simulink model "wheels2fin"  (R2014a)
settings: Solver=ode15s  StartTime=0.0  StopTime=20  MaxStep=.01  RelTol=1e-3  AbsTol=1e-6  EnableMultiTasking=on
PreLoadFcn:
  | % Load initialization data
  | 
  | sldemo_absdata;
StopFcn:
  | if exist ('wheels2_output')
  |   wheels2plots;
  | end
undefined symbols (not defined in the file): ctrl, mu, slip
libraries: fl_lib x5, sh_lib x3, nesl_utility x3, aerospace x1, powerlib_meascontrol x1, simulink x1
CloseFcn:
  | % Close the plots that are still open
  | h = findobj(0, 'Name', 'ABS Speeds');
  | if ~isempty(h),
  |   close(h);
  | end;
  | 
  | h = findobj(0, 'Name', 'ABS Slip');
  | if ~isempty(h),
  |   close(h);
  | end;
  | 
  | % Clear initial conditions data to avoid cluttering the workspace
  | 
  | clear g v0 Rr Kf m PBmax TB I slip mu ctrl h;
Description:
  | Modeling an Anti-Lock Braking System (ABS)
  | 
  | *Summary*
  | 
  | This example describes a simple model for an Anti-Lock Braking System
  | (ABS). The model simulates the dynamic behavior of a vehicle
  | under hard braking conditions. The model represents a single wheel, which
  | may be replicated a number of times to create a model for a multi-wheel
  | vehicle.
  | 
  | This model uses the signal logging feature in Simulink(R). You log signals to the
  | MATLAB(R) workspace where you can analyze and view them. You can view
  | the code in sldemo_absbrakeplots.m to see how this is done.
  | 
  | In this model, the wheel speed is calculated in a separate component
  | named sldemo_wheelspeed_absbrake.
  | This component is then referenced using a Model block.  Note that both the
  | top model and the referenced model use a variable step solver, so Simulink
  | will track zero-crossings in the referenced model.
settings Model: FPTRunName=Active  ExtModeTrigMode=oneshot  ExtModeTrigDuration=8  ExtModeArmWhenConnect=off  ExtModeAutoUpdateStatusClock=off  Creator=The MathWorks, Inc.  LastModifiedBy=Abi
settings SolverCC: AutoScaleAbsTol=off
settings DataIOCC: LimitDataPoints=off  SaveOutput=off  SaveTime=off  TimeSaveName=time  SignalLoggingName=sldemo_absbrake_output
settings OptimizationCC: DefaultUnderspecifiedDataType=single  EnhancedBackFolding=on  PassReuseOutputArgsAs=Individual arguments  ExpressionDepthLimit=2147483647  InitFltsAndDblsToZero=on  LifeSpan=auto  MaxStackSize=512  BufferReusableBoundary=off  SimCompilerOptimization=off  OptimizeBlockOrder=speed  DifferentSizesBufferReuse=on  OptimizationCustomize=off
settings DebuggingCC: SaveWithParameterizedLinksMsg=none  MergeDetectMultiDrivingBlocksExec=error  SolverPrmCheckMsg=none  MultiTaskDSMMsg=warning  SigSpecEnsureSampleTimeMsg=none  IntegerOverflowMsg=none  ParameterTunabilityLossMsg=error  FcnCallInpInsideContextMsg=warning  FrameProcessingCompatibilityMsg=error  BusObjectLabelMismatch=none  AllowSymbolicDim=off  StateNameClashWarn=warning  SFExecutionAtInitializationDiag=none  IntegerSaturationMsg=none  ArithmeticOperatorsInVariantConditions=warning
settings HardwareCC: ProdBitPerChar=16  ProdBitPerInt=16  ProdBitPerSizeT=32  ProdBitPerPtrDiffT=32  ProdLargestAtomicInteger=Integer  ProdIntDivRoundTo=Zero  ProdEndianess=LittleEndian  ProdWordSize=16  ProdLongLongMode=on  ProdHWDeviceType=Texas Instruments->C2000  TargetBitPerPointer=64  TargetBitPerSizeT=64  TargetBitPerPtrDiffT=64  TargetLongLongMode=on  TargetIntDivRoundTo=Zero  TargetEndianess=LittleEndian  TargetWordSize=64  TargetHWDeviceType=MATLAB Host
settings ModelReferenceCC: UpdateModelReferenceTargets=IfOutOfDate
settings SFSimCC: MATLABDynamicMemAlloc=off
settings RTWCC: SystemTargetFile=ert.tlc  HardwareBoard=TI Piccolo F28069M LaunchPad  TLCOptions=-aInlineSetEventsForThisBaseRateFcn=TLC_FALSE -aSuppressMultiTaskScheduler=TLC_FALSE -aRateBasedStepFcn=1  TemplateMakefile=ert_default_tmf  Description=Embedded Coder  GenerateReport=on  Toolchain=Texas Instruments Code Composer Studio (C2000)  IncludeHyperlinkInReport=on  LaunchReport=on  GenerateTraceInfo=on  GenerateTraceReport=on  GenerateTraceReportSl=on  GenerateTraceReportSf=on  GenerateTraceReportEml=on  RTWCompilerOptimization=off
settings CodeAppCC: ForceParamTrailComments=on  IgnoreCustomStorageClasses=off  OperatorAnnotations=on  SimulinkDataObjDesc=on  SFDataObjDesc=on  InsertBlockDesc=on
settings ERTTargetCC: CodeReplacementLibrary=TI C28x  MultiwordLength=256  GenerateSampleERTMain=off  ParMdlRefBuildCompliant=on  CompOptLevelCompliant=on  ConcurrentExecutionCompliant=on  ModelStepFunctionPrototypeControlCompliant=on  CPPClassGenCompliant=on  InlinedParameterPlacement=Hierarchical  ConvertIfToSwitch=on  SuppressUnreachableDefaultCases=on
settings ConfigComp: CovMetricSettings=dw  CovHtmlReporting=on  CovSaveCumulativeToWorkspaceVar=on  CovSaveSingleToWorkspaceVar=on  CovExternalEMLEnable=off  CovSFcnEnable=off

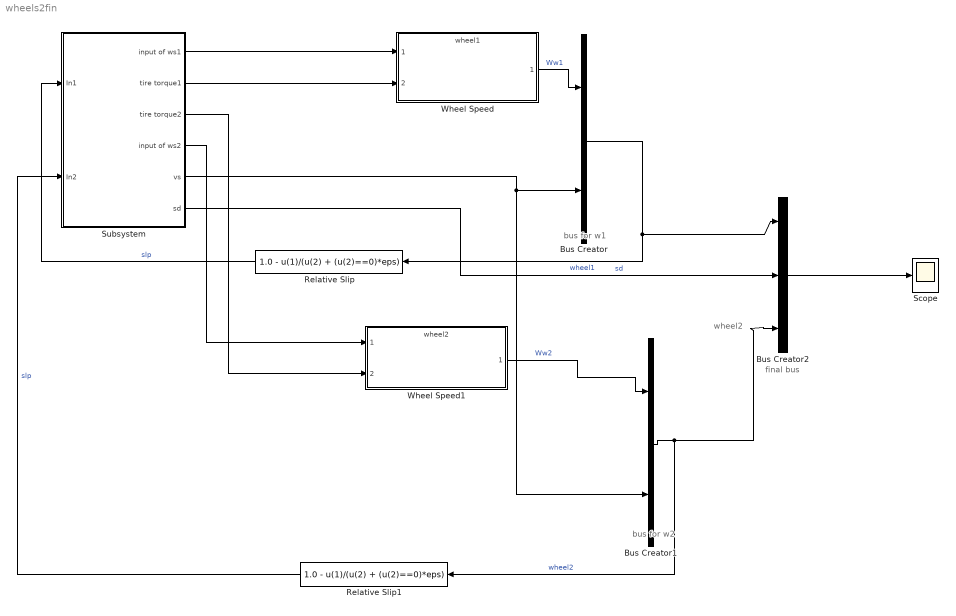
== system wheels2fin ==
  note: bus for w2
  note: bus for w1
  note: final bus
  note: wheel2
  Bus Creator2 : BusCreator  Inputs=3
  Bus Creator : BusCreator  Inputs=2
  Bus Creator1 : BusCreator  Inputs=2
  Relative Slip : Fcn  Expr=1.0 - u(1)/(u(2) + (u(2)==0)*eps)
  Relative Slip1 : Fcn  Expr=1.0 - u(1)/(u(2) + (u(2)==0)*eps)
  Scope : Scope
  Subsystem : Subsystem
  Wheel Speed : ModelReference  ModelNameDialog=wheel1.slx  SimulationMode=Normal  ModelReferenceVersion=1.65  CopyOfModelName=wheel1.slx  DefaultDataLogging=on
  Wheel Speed1 : ModelReference  ModelNameDialog=wheel2.slx  SimulationMode=Normal  ModelReferenceVersion=1.65  CopyOfModelName=wheel2.slx  DefaultDataLogging=on
  wires:
  Wheel Speed/1 -> Bus Creator/1  "Ww1"
  Relative Slip/1 -> Subsystem/1(In1)  "slp"
  Bus Creator/1 -> Relative Slip/1, Bus Creator2/1  "wheel1"
  Wheel Speed1/1 -> Bus Creator1/1  "Ww2"
  Bus Creator1/1 -> Bus Creator2/3, Relative Slip1/1  "wheel2"
  Relative Slip1/1 -> Subsystem/2(In2)  "slp"
  Subsystem/1(input of ws1) -> Wheel Speed/1
  Subsystem/2("tire torque1 ") -> Wheel Speed/2
  Subsystem/3(tire torque2) -> Wheel Speed1/2
  Subsystem/5(vs) -> Bus Creator1/2, Bus Creator/2
  Subsystem/4(input of ws2) -> Wheel Speed1/1
  Bus Creator2/1 -> Scope/1
  Subsystem/6("sd ") -> Bus Creator2/2  "sd"

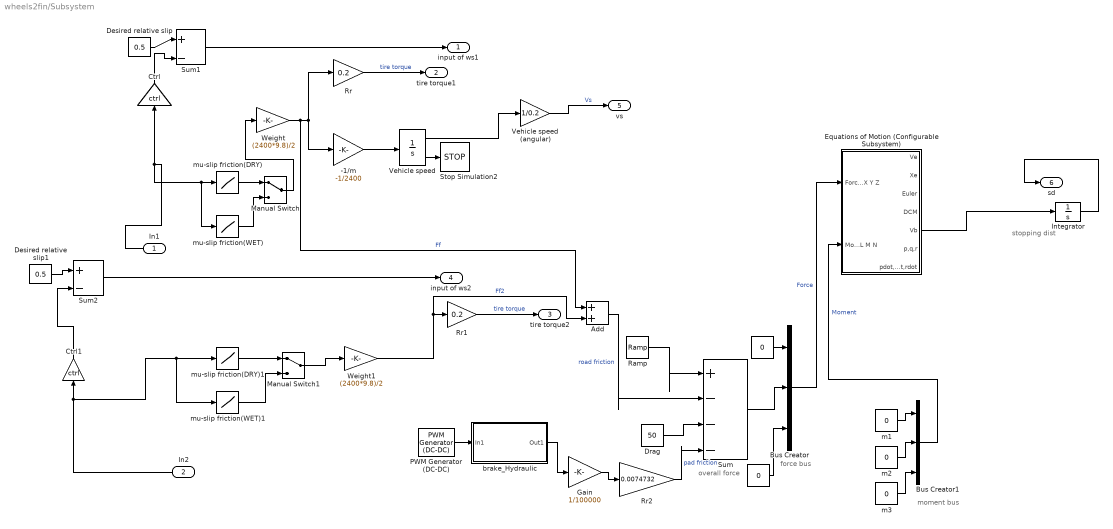
== system wheels2fin/Subsystem ==
  note: moment bus
  note: force bus
  note: stopping dist
  note: overall force
  In1 : Inport
  In2 : Inport  Port=2
  " " : Constant  Value=0
  " " : Constant  Value=0
  -1/m : Gain  Gain=-1/2400  SaturateOnIntegerOverflow=on  OutDataTypeStr=Inherit: Same as input  ParamDataTypeStr=Inherit: Same as input
  Add : Sum
  Bus Creator : BusCreator  Inputs=3
  Bus Creator1 : BusCreator  Inputs=3
  Ctrl : Gain  Gain=ctrl  SaturateOnIntegerOverflow=on  OutDataTypeStr=Inherit: Same as input  ParamDataTypeStr=Inherit: Same as input
  Ctrl1 : Gain  Gain=ctrl  SaturateOnIntegerOverflow=on  OutDataTypeStr=Inherit: Same as input  ParamDataTypeStr=Inherit: Same as input
  Desired relative slip : Constant  Value=0.5
  Desired relative slip1 : Constant  Value=0.5
  Drag : Constant  Value=50
  Equations of Motion (Configurable Subsystem) : Subsystem  BlockChoice=Euler Angles
      link override Euler Angles: Mass=2400
      settings: AttributesFormatString=%<BlockChoice>  MemberBlocks=Euler Angles,Quaternions
      settings: TemplateBlock=|
      | aerospace/6DoF/Equations of Motion
      | (Configurable Subsystem)
  Gain : Gain  Gain=1/100000
  Integrator : Integrator
  Manual Switch : ManualSwitch
  Manual Switch1 : ManualSwitch
  PWM Generator (DC-DC) : powerlib_meascontrol/Pulse & Signal Generators/PWM Generator (DC-DC)  Fsw=5000  Ts=0
  Ramp : simulink/Sources/Ramp  slope=1  start=0  X0=0
  Rr : Gain  Gain=0.2  SaturateOnIntegerOverflow=on  OutDataTypeStr=Inherit: Same as input  ParamDataTypeStr=Inherit: Same as input
  Rr1 : Gain  Gain=0.2  SaturateOnIntegerOverflow=on  OutDataTypeStr=Inherit: Same as input  ParamDataTypeStr=Inherit: Same as input
  Rr2 : Gain  Gain=0.0074732  SaturateOnIntegerOverflow=on  OutDataTypeStr=Inherit: Same as input  ParamDataTypeStr=Inherit: Same as input
  Stop Simulation2 : Stop
  Sum : Sum  Inputs=|+---
  Sum1 : Sum  Inputs=|+-  SaturateOnIntegerOverflow=on  InputSameDT=on  OutDataTypeStr=Inherit: Same as first input
  Sum2 : Sum  Inputs=|+-  SaturateOnIntegerOverflow=on  InputSameDT=on  OutDataTypeStr=Inherit: Same as first input
  Vehicle speed : Integrator  UpperSaturationLimit=1000  LowerSaturationLimit=0  ShowSaturationPort=on
  Vehicle speed (angular) : Gain  Gain=1/0.2  SaturateOnIntegerOverflow=on  OutDataTypeStr=Inherit: Same as input  ParamDataTypeStr=Inherit: Same as input
  Weight : Gain  Gain=(2400*9.8)/2  SaturateOnIntegerOverflow=on  OutDataTypeStr=Inherit: Same as input  ParamDataTypeStr=Inherit: Same as input
  Weight1 : Gain  Gain=(2400*9.8)/2  SaturateOnIntegerOverflow=on  OutDataTypeStr=Inherit: Same as input  ParamDataTypeStr=Inherit: Same as input
  "brake_Hydraulic " : Subsystem
  m1 : Constant  Value=0
  "m2 " : Constant  Value=0
  m3 : Constant  Value=0
  mu-slip friction(DRY) : Lookup_n-D  NumberOfTableDimensions=1  BreakpointsForDimension1=slip  Table=mu  SaturateOnIntegerOverflow=on  InputSameDT=on
  mu-slip friction(DRY)1 : Lookup_n-D  NumberOfTableDimensions=1  BreakpointsForDimension1=slip  Table=mu  SaturateOnIntegerOverflow=on  InputSameDT=on
  mu-slip friction(WET) : Lookup_n-D  NumberOfTableDimensions=1  BreakpointsForDimension1=slip  Table=mu  SaturateOnIntegerOverflow=on  InputSameDT=on
  mu-slip friction(WET)1 : Lookup_n-D  NumberOfTableDimensions=1  BreakpointsForDimension1=slip  Table=mu  SaturateOnIntegerOverflow=on  InputSameDT=on
  input of ws1 : Outport
  "tire torque1 " : Outport  Port=2
  tire torque2 : Outport  Port=3
  input of ws2 : Outport  Port=4
  vs : Outport  Port=5
  "sd " : Outport  Port=6
  wires:
  Weight/1 -> Add/1, -1/m/1, Rr/1  "Ff"
  Rr/1 -> "tire torque1 "/1  "tire torque"
  Sum1/1 -> input of ws1/1
  -1/m/1 -> Vehicle speed/1
  Desired relative slip/1 -> Sum1/1
  Ctrl/1 -> Sum1/2
  Vehicle speed/2 -> Stop Simulation2/1
  Vehicle speed/1 -> Vehicle speed (angular)/1
  Vehicle speed (angular)/1 -> vs/1  "Vs"
  Desired relative slip1/1 -> Sum2/1
  Sum2/1 -> input of ws2/1
  Ctrl1/1 -> Sum2/2
  Rr1/1 -> tire torque2/1  "tire torque"
  Weight1/1 -> Add/2, Rr1/1  "Ff2"
  "brake_Hydraulic "/1(Out1) -> Gain/1
  Ramp/1 -> Sum/1
  Add/1 -> Sum/2  "road friction"
  Drag/1 -> Sum/3
  " "/1 -> Bus Creator/3
  m3/1 -> Bus Creator1/3
  "m2 "/1 -> Bus Creator1/2
  m1/1 -> Bus Creator1/1
  Bus Creator1/1 -> Equations of Motion (Configurable Subsystem)/2(Moments L M N)  "Moment"
  Integrator/1 -> "sd "/1
  Bus Creator/1 -> Equations of Motion (Configurable Subsystem)/1(Forces X Y Z)  "Force"
  Equations of Motion (Configurable Subsystem)/5(Vb) -> Integrator/1
  " "/1 -> Bus Creator/1
  Sum/1 -> Bus Creator/2
  Gain/1 -> Rr2/1
  Rr2/1 -> Sum/4  "pad friction"
  In2/1 -> mu-slip friction(WET)1/1, mu-slip friction(DRY)1/1, Ctrl1/1
  In1/1 -> Ctrl/1, mu-slip friction(WET)/1, mu-slip friction(DRY)/1
  mu-slip friction(DRY)/1 -> Manual Switch/1
  mu-slip friction(WET)/1 -> Manual Switch/2
  Manual Switch/1 -> Weight/1
  mu-slip friction(DRY)1/1 -> Manual Switch1/1
  mu-slip friction(WET)1/1 -> Manual Switch1/2
  Manual Switch1/1 -> Weight1/1
  PWM Generator (DC-DC)/1 -> "brake_Hydraulic "/1(In1)

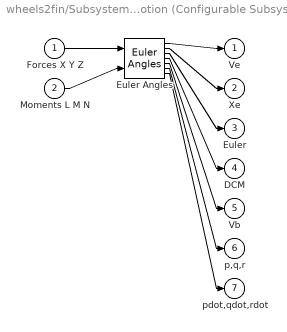
== system wheels2fin/Subsystem/Equations of Motion (Configurable Subsystem) ==
  Forces X Y Z : Inport
  Moments L M N : Inport  Port=2
  Euler Angles : aerospace/6DoF/Euler Angles  xme_0=[0 0 0]  Vm_0=[0 0 0]  eul_0=[0 0 0]  pm_0=[0 0 0]  Mass=2400  Inertia=eye(3)
  Ve : Outport
  Xe : Outport  Port=2
  Euler : Outport  Port=3
  DCM : Outport  Port=4
  Vb : Outport  Port=5
  p,q,r : Outport  Port=6
  pdot,qdot,rdot : Outport  Port=7
  wires:
  Forces X Y Z/1 -> Euler Angles/1
  Moments L M N/1 -> Euler Angles/2
  Euler Angles/1 -> Ve/1
  Euler Angles/2 -> Xe/1
  Euler Angles/3 -> Euler/1
  Euler Angles/4 -> DCM/1
  Euler Angles/5 -> Vb/1
  Euler Angles/6 -> p,q,r/1
  Euler Angles/7 -> pdot,qdot,rdot/1

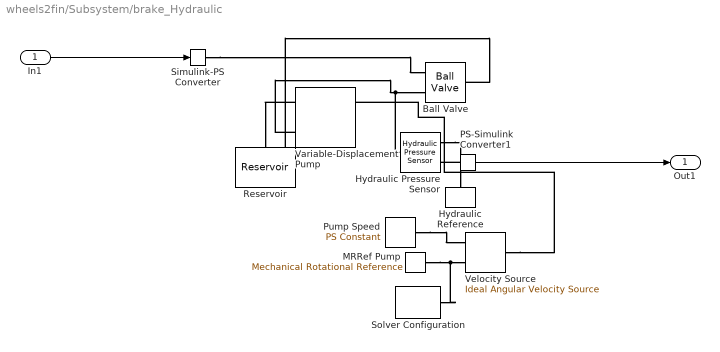
== system wheels2fin/Subsystem/brake_Hydraulic  ==
  In1 : Inport
  Ball Valve : sh_lib/Valves/Flow Control Valves/Ball Valve  d_ball=0.01 m  d_orif=0.005 m  x_0=0 m  C_d=0.65  Re_cr=10  A_leak=1e-12 m^2
  Hydraulic Pressure Sensor : fl_lib/Hydraulic/Hydraulic Sensors/Hydraulic Pressure Sensor
  Hydraulic Reference : fl_lib/Hydraulic/Hydraulic Elements/Hydraulic Reference
  MRRef Pump : fl_lib/Mechanical/Rotational Elements/Mechanical Rotational Reference  Tag=Factory Generic
  PS-Simulink Converter1 : nesl_utility/PS-Simulink Converter  PhysicalDomain=network_engine_domain  SubClassName=ps_output  LeftPortType=input  RightPortType=output  PseudoPeriodic=off  Frequencies=[]  Unit=1  AffineConversion=off
  Pump Speed : fl_lib/Physical Signals/Sources/PS Constant  constant=1
  Reservoir : sh_lib/Hydraulic Utilities/Reservoir  press=0 Pa  init_volume=0.02 m^3  ret_diam=0.02 m  loss_coeff=1  Re_lam=15  area=1e-4 m^2  p_cr=1e-5 Pa
  Simulink-PS Converter : nesl_utility/Simulink-PS Converter  PhysicalDomain=network_engine_domain  SubClassName=ps_input  LeftPortType=input  RightPortType=output  PseudoPeriodic=off  Frequencies=[]  NoiseDistribution=none  NoiseParameters=[]  Unit=1  AffineConversion=off  InputFiltering=off  SimscapeFilterOrder=1  InputFilterTimeConstant=0.001  UdotUserProvided=1
  Solver Configuration : nesl_utility/Solver Configuration  PhysicalDomain=network_engine_domain  SubClassName=solver  LeftPortType=input  RightPortType=generic  Accelerate=off  Tones=[]  Harmonics=[]  SimulateNoise=off  Profile=off  UseLocalSampling=off  EnableSwitchedLinearOptims=on  FrequencyDomain=off  UseCCode=off  RelTol=0.001  AbsTol=1e-06  MinStep=1e-09  ToWorkspace=off  DoDC=off  ResidualTolerance=1e-09  UseLocalSolver=off  LocalSolverChoice=NE_BACKWARD_EULER_ADVANCER  LocalSolverSampleTime=0.001  DoFixedCost=off  MaxNonlinIter=3  MaxModeIter=2  LinearAlgebra=Sparse  DelaysMemoryBudget=1024  AutomaticFiltering=on  FilteringTimeConstant=0.001
  Variable-Displacement Pump : sh_lib/Pumps and Motors/Variable-Displacement Pump  mdl_type=1  D_max=5e-6 m^3/rad  stroke_max=0.005 m  displ_tab=[- 5e-6, - 3e-6, 0, 3e-6, 5e-6] m^3/rad  cntrl_mem_tab=[- 7.5e-3, - 2.5e-3, 0, 2.5e-3, 7.5e-3] m  interp_method=1  extrap_method=1  efficiency_vol=0.85  efficiency_tot=0.75  pr_nominal=100e5 Pa  w_nominal=188 rad/s  visc_nominal=18 cSt  dens_nominal=900 kg/m^3  k_leak=1e-11 m^3/s/Pa  efficiency_mech=0.7
  Velocity Source : fl_lib/Mechanical/Mechanical Sources/Ideal Angular Velocity Source  Tag=Factory Generic
  Out1 : Outport
  wires:
  PS-Simulink Converter1/1 -> Out1/1
  In1/1 -> Simulink-PS Converter/1
  connections:
  Reservoir/LConn3 -- Ball Valve/RConn1
  Simulink-PS Converter/RConn1 -- Ball Valve/LConn1
  Hydraulic Pressure Sensor/RConn1 -- Hydraulic Reference/LConn1
  PS-Simulink Converter1/LConn1 -- Hydraulic Pressure Sensor/RConn2
  Variable-Displacement Pump/RConn2 -- Reservoir/LConn2
  Variable-Displacement Pump/RConn1 -- Hydraulic Pressure Sensor/LConn1 -- Ball Valve/LConn2
  Velocity Source/RConn2 -- MRRef Pump/LConn1 -- Solver Configuration/RConn1
  Pump Speed/RConn1 -- Velocity Source/RConn1
  Velocity Source/LConn1 -- Variable-Displacement Pump/LConn2
